simulink model "inf_horiz_sml"  (Simulink 8.7)
settings: Solver=ode45  StartTime=0.0  StopTime=10  MaxStep=.01  RelTol=1e-3
values from neighbouring files (symbols this model uses):
  J = x0'*P*x0    [inf_horiz.m]
  Q = [2 1; 1 4]    [Riccati_sol2.m]    (also in file_for_LQR_EX.m = [100 0 ; 0 0]; inf_horiz.m = [10 0; 0 2000])
  R = 1/2    (= 0.5)    [Riccati_sol2.m]    (also in file_for_LQR_EX.m = 10; inf_horiz.m = 1)
  x1 = 10    [inf_horiz.m]
  x2 = 10    [inf_horiz.m]
undefined symbols (not defined in the file or in its folder): K
libraries: simulink x1
settings Model: Creator=Thomas Chmielewski  LastModifiedBy=DR_C
settings DataIOCC: SignalLoggingSaveFormat=ModelDataLogs
settings OptimizationCC: ExpressionDepthLimit=2147483647
settings DebuggingCC: SolverPrmCheckMsg=warning  FcnCallInpInsideContextMsg=UseLocalSettings  StateNameClashWarn=warning
settings GRTTargetCC: CombineOutputUpdateFcns=off  GRTInterface=on

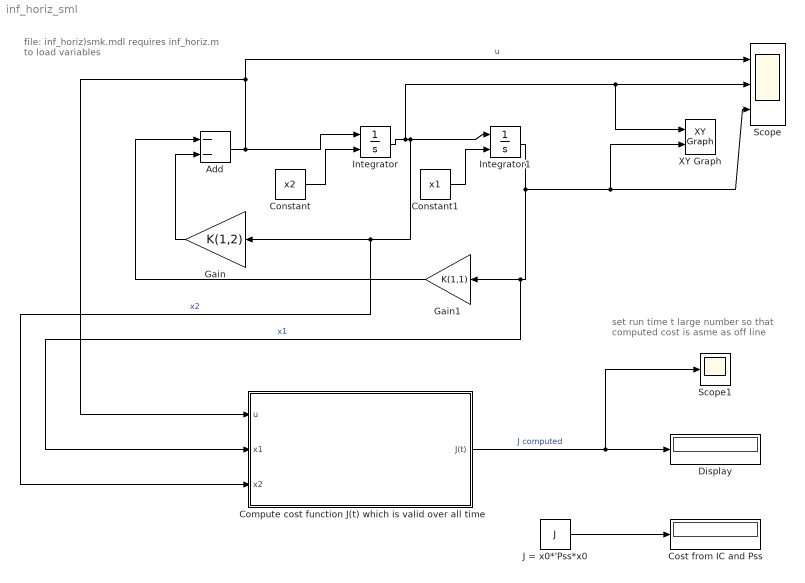
== system inf_horiz_sml ==
  note: set run time t large number so that
      | computed cost is asme as off line
  note: file:  inf_horiz)smk.mdl
      | requires inf_horiz.m to load variables
  Add : Sum  Inputs=--
  Compute cost function J(t) which is valid over all time : Subsystem
  Constant : Constant  Value=x2
  Constant1 : Constant  Value=x1
  Cost from IC and Pss : Display
  Display : Display
  Gain : Gain  Gain=K(1,2)
  Gain1 : Gain  Gain=K(1,1)
  Integrator : Integrator  InitialConditionSource=external
  Integrator1 : Integrator  InitialConditionSource=external
  J = x0*'Pss*x0 : Constant  Value=J
  Scope : Scope  NumInputPorts=3
  Scope1 : Scope
  XY Graph : simulink/Sinks/XY Graph  xmin=-10  xmax=10  ymin=-10  ymax=10  st=-1
  wires:
  Add/1 -> Integrator/1, Scope/1, Compute cost function J(t) which is valid over all time/1(u)  "u"
  Integrator/1 -> Integrator1/1, Gain/1, Compute cost function J(t) which is valid over all time/3(x2), Scope/2, XY Graph/1  "x2"
  Integrator1/1 -> Gain1/1, Compute cost function J(t) which is valid over all time/2(x1), Scope/3, XY Graph/2  "x1"
  Gain/1 -> Add/2
  Gain1/1 -> Add/1
  Constant1/1 -> Integrator1/2
  Constant/1 -> Integrator/2
  Compute cost function J(t) which is valid over all time/1(J(t)) -> Display/1, Scope1/1  "J computed"
  J = x0*'Pss*x0/1 -> Cost from IC and Pss/1

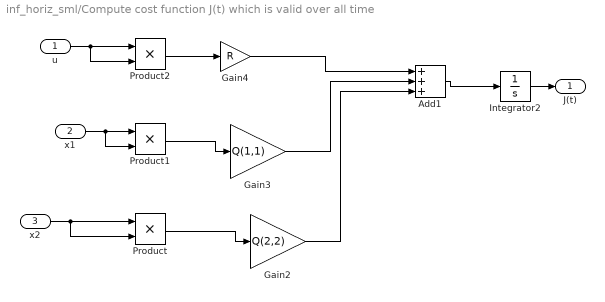
== system inf_horiz_sml/Compute cost function J(t) which is valid over all time ==
  u : Inport
  x1 : Inport  Port=2
  x2 : Inport  Port=3
  Add1 : Sum  Inputs=+++
  Gain2 : Gain  Gain=Q(2,2)
  Gain3 : Gain  Gain=Q(1,1)
  Gain4 : Gain  Gain=R
  Integrator2 : Integrator
  Product : Product  RndMeth=Zero
  Product1 : Product  RndMeth=Zero
  Product2 : Product  RndMeth=Zero
  J(t) : Outport
  wires:
  Add1/1 -> Integrator2/1
  Product2/1 -> Gain4/1
  Gain4/1 -> Add1/1
  Product1/1 -> Gain3/1
  Gain3/1 -> Add1/2
  Product/1 -> Gain2/1
  Gain2/1 -> Add1/3
  u/1 -> Product2/1, Product2/2
  x1/1 -> Product1/1, Product1/2
  x2/1 -> Product/1, Product/2
  Integrator2/1 -> J(t)/1
